simulink model "reactor_nonlinear_vs_linear_model_simulation"  (Simulink 10.2)
settings: Solver=ode15s  StartTime=0.0  StopTime=100  RelTol=1e-3  EnableMultiTasking=on
values from neighbouring files (symbols this model uses):
  A_linearized = [df1_dx1 df1_dx2 df1_dx3 df1_dx4;     df2_dx1 df2_dx2 df2_dx3 df2_dx4;     df3_dx1 df3_dx2 df3_dx3 df3_dx4;     df4_dx1 df4_dx2 df4_dx3 df4_dx4]    [assignment_q2.m]
  B_linearized = [df1_du1 df1_du2;     df2_du1 df2_du2;     df3_du1 df3_du2;     df4_du1 df4_du2]    [assignment_q2.m]
  C_A_steady = x_ss(1)    [assignment_q2.m]
  C_B_steady = x_ss(2)    [assignment_q2.m]
  C_linearized = eye(4)    [assignment_q2.m]
  T_J_steady = x_ss(4)    [assignment_q2.m]
  T_R_steady = x_ss(3)    [assignment_q2.m]
  u_s = [Fr_ss Qj_ss]    [assignment_q2.m]
  u_s_part4_1 = 0.9*u_s    [assignment_q2.m]
  x0 = [-5; 0]    [assignment_q1.m]    (also in assignment_q2.m = [0; 0; 387.05; 387.05]; reactor_nonlinear_sfcn.m = x0_7_1)
settings Model: Creator=LemoineR  LastModifiedBy=mbatu
settings DataIOCC: LimitDataPoints=on
settings OptimizationCC: ExpressionDepthLimit=2147483647
settings DebuggingCC: SolverPrmCheckMsg=warning  StateNameClashWarn=warning

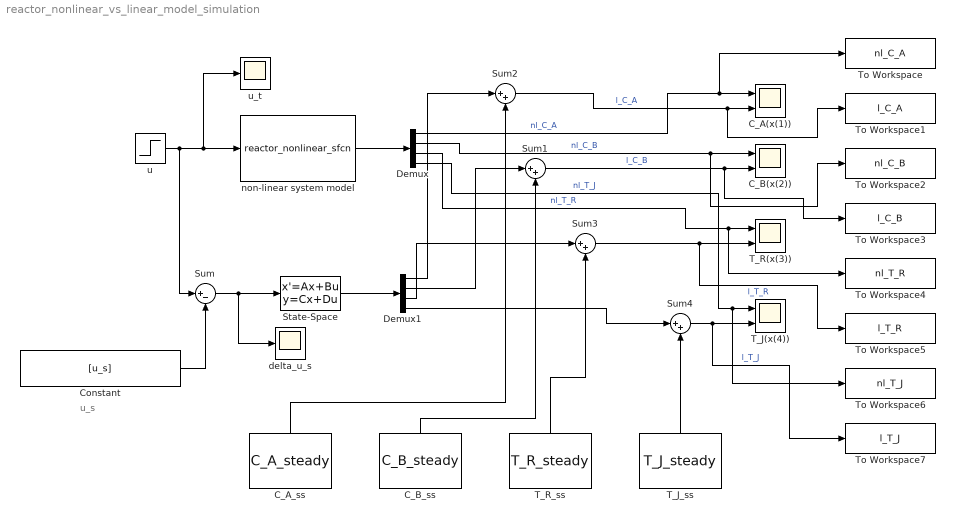
== system reactor_nonlinear_vs_linear_model_simulation ==
  note: u_s
  C_A(x(1)) : Scope  NumInputPorts=2
  "C_A_ss " : Constant  Value=C_A_steady
  C_B(x(2)) : Scope  NumInputPorts=2
  C_B_ss : Constant  Value=C_B_steady
  Constant : Constant  Value=[u_s]
  Demux : Demux
  Demux1 : Demux
  State-Space : StateSpace  A=A_linearized  B=B_linearized  C=C_linearized  D=[0 0; 0 0; 0 0; 0 0];  InitialCondition=x0
  Sum : Sum  Inputs=|+-
  Sum{1..4} (4 alike) : Sum  Inputs=|++
  T_J(x(4)) : Scope  NumInputPorts=2
  T_J_ss : Constant  Value=T_J_steady
  T_R(x(3)) : Scope  NumInputPorts=2
  T_R_ss : Constant  Value=T_R_steady
  To Workspace : ToWorkspace  VariableName=nl_C_A  SampleTime=-1
  To Workspace1 : ToWorkspace  VariableName=l_C_A  SampleTime=-1
  To Workspace2 : ToWorkspace  VariableName=nl_C_B  SampleTime=-1
  To Workspace3 : ToWorkspace  VariableName=l_C_B  SampleTime=-1
  To Workspace4 : ToWorkspace  VariableName=nl_T_R  SampleTime=-1
  To Workspace5 : ToWorkspace  VariableName=l_T_R  SampleTime=-1
  To Workspace6 : ToWorkspace  VariableName=nl_T_J  SampleTime=-1
  To Workspace7 : ToWorkspace  VariableName=l_T_J  SampleTime=-1
  delta_u_s : Scope
  non-linear system model : S-Function  FunctionName=reactor_nonlinear_sfcn  SFunctionDeploymentMode=off  EnableBusSupport=off
  u : Step  Time=0  Before=u_s_part4_1  After=u_s_part4_1  SampleTime=0
  u_t : Scope
  wires:
  u/1 -> u_t/1, non-linear system model/1, Sum/1
  non-linear system model/1 -> Demux/1
  Sum/1 -> State-Space/1, delta_u_s/1
  Constant/1 -> Sum/2
  State-Space/1 -> Demux1/1
  Demux/1 -> To Workspace/1, C_A(x(1))/1  "nl_C_A"
  Demux/2 -> To Workspace2/1, C_B(x(2))/1  "nl_C_B"
  Demux/3 -> To Workspace4/1, T_R(x(3))/1  "nl_T_R"
  Demux/4 -> To Workspace6/1, T_J(x(4))/1  "nl_T_J"
  Sum2/1 -> To Workspace1/1, C_A(x(1))/2  "l_C_A"
  Demux1/1 -> Sum2/1
  "C_A_ss "/1 -> Sum2/2
  Sum1/1 -> To Workspace3/1, C_B(x(2))/2  "l_C_B"
  Demux1/2 -> Sum1/1
  C_B_ss/1 -> Sum1/2
  Sum3/1 -> To Workspace5/1, T_R(x(3))/2  "l_T_R"
  Demux1/3 -> Sum3/1
  T_R_ss/1 -> Sum3/2
  Sum4/1 -> To Workspace7/1, T_J(x(4))/2  "l_T_J"
  T_J_ss/1 -> Sum4/2
  Demux1/4 -> Sum4/1
